simulink model "AAI_Pacemaker"  (R2022a)
settings: Solver=FixedStepAuto  StartTime=0.0  StopTime=10.0  FixedStep=1e-3  RelTol=1e-3  EnableMultiTasking=on
settings Model: ExtModeTrigDuration=5  Creator=vinee  LastModifiedBy=yajatsharma
settings SolverCC: AlgebraicLoopSolver=TrustRegion
settings OptimizationCC: EnhancedBackFolding=on  PassReuseOutputArgsAs=Individual arguments  ZeroExternalMemoryAtStartup=off  ZeroInternalMemoryAtStartup=off  MaxStackSize=64  OptimizeBlockOrder=speed  DifferentSizesBufferReuse=on  OptimizationCustomize=off  EfficientTunableParamExpr=on
settings DebuggingCC: ParameterTunabilityLossMsg=error  UnconnectedInputMsg=warning  UnconnectedOutputMsg=warning  UnconnectedLineMsg=warning  SFMachineParentedDataDiag=warning
settings HardwareCC: ProdBitPerPointer=32  ProdBitPerSizeT=32  ProdBitPerPtrDiffT=32  ProdLargestAtomicInteger=Long  ProdLargestAtomicFloat=Double  ProdWordSize=32  ProdHWDeviceType=ARM Compatible->ARM Cortex
settings SFSimCC: MATLABDynamicMemAlloc=off
settings RTWCC: SystemTargetFile=ert.tlc  HardwareBoard=NXP FRDM-K64F  TLCOptions="-aInlineSetEventsForThisBaseRateFcn=TLC_FALSE -aSuppressMultiTaskScheduler=TLC_FALSE  -aRateBasedStepFcn=0"  TemplateMakefile=ert_default_tmf  Toolchain=GNU Tools for ARM Embedded Processors
settings CodeAppCC: ForceParamTrailComments=on  IgnoreCustomStorageClasses=off  OperatorAnnotations=on  SimulinkDataObjDesc=on  SFDataObjDesc=on  InsertBlockDesc=on

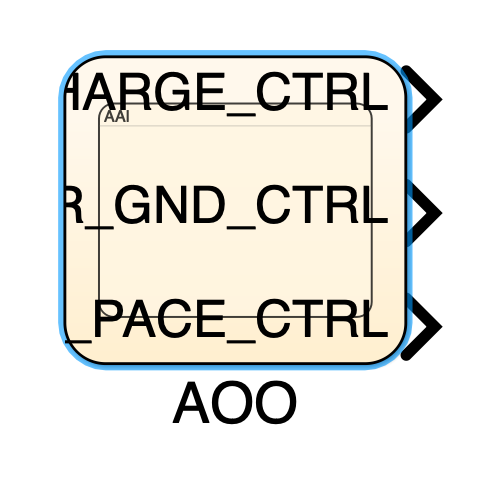
[thumbnail: Simulink's stored preview of the top-level diagram]
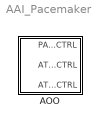
== system AAI_Pacemaker ==
  AOO : Stateflow chart  TreatAsAtomicUnit=on

== stateflow chart AAI_Pacemaker/AOO ==
  state AAI
    entry:
    Z_ATR_CTRL = 0;
    Z_VENT_CTRL =0;
    ATR_GND_CTRL = 0;
    ATR_PACE_CTRL =0;
    PACE_GND_CTRL = 1;
    PACING_REF_PWM = A_AMP;
    state DISCHARGE_C22_PACE_ATR
      entry:
      PACE_CHARGE_CTRL = 0;
      ATR_PACE_CTRL = 1;
      ATR_GND_CTRL = 0;
    state CHARGE_C22
      entry:
      ATR_PACE_CTRL = 0;
      ATR_GND_CTRL = 1;
      PACE_CHARGE_CTRL =1;
    state REFRACTORY_PERIOD
      entry:
      PACE_CHARGE_CTRL=1;
      ATR_PACE_CTRL=0;
      ATR_GND_CTRL=1;
    (default) -> CHARGE_C22
    CHARGE_C22 -> DISCHARGE_C22_PACE_ATR : [after(APW,msec)]
    DISCHARGE_C22_PACE_ATR -> REFRACTORY_PERIOD : [after(APW,msec)]
    REFRACTORY_PERIOD -> CHARGE_C22 : [after(APW,msec)]
  data: PACE_CHARGE_CTRL output; ATR_GND_CTRL output; ATR_PACE_CTRL output
